simulink model "sistema_doble_pendulo"  (R2022b)
settings: Solver=VariableStepAuto  StartTime=0.0  StopTime=10  MaxStep=.00001  RelTol=1e-3
undefined symbols (not defined in the file): g, l1, l2, m1, m2
settings Model: Creator=bryan  LastModifiedBy=bryan

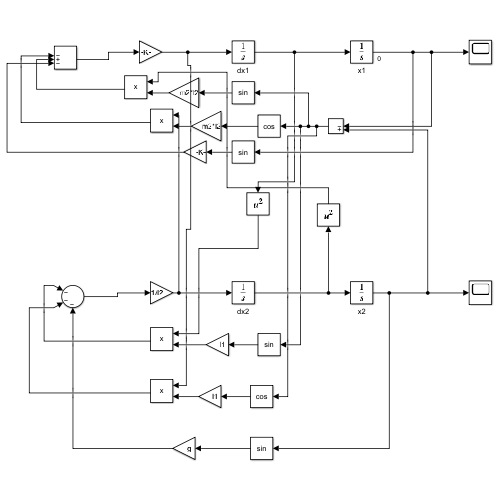
[thumbnail: Simulink's stored preview of the top-level diagram]
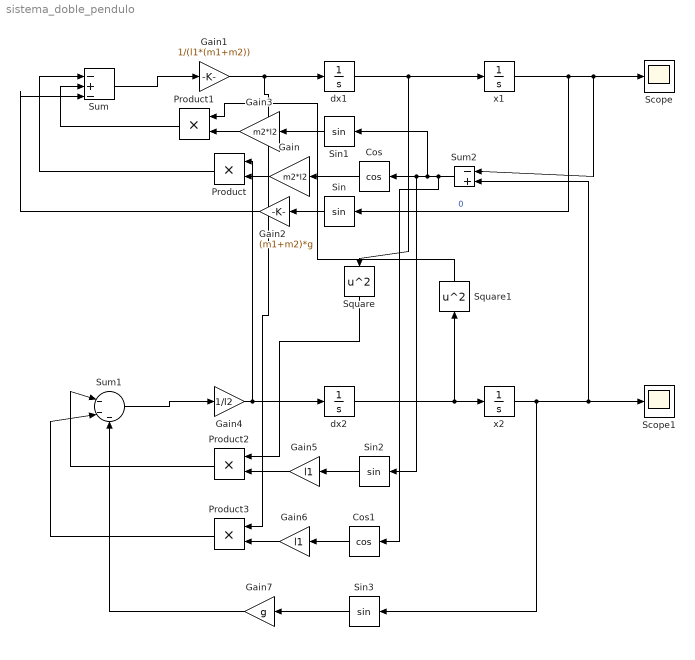
== system sistema_doble_pendulo ==
  Cos : Trigonometry  Operator=cos
  Cos1 : Trigonometry  Operator=cos
  Gain : Gain  Gain=m2*l2
  Gain1 : Gain  Gain=1/(l1*(m1+m2))
  Gain2 : Gain  Gain=(m1+m2)*g
  Gain3 : Gain  Gain=m2*l2
  Gain4 : Gain  Gain=1/l2
  Gain5 : Gain  Gain=l1
  Gain6 : Gain  Gain=l1
  Gain7 : Gain  Gain=g
  Product{,1..3} (4 alike) : Product
  Scope : Scope
  Scope1 : Scope
  Sin{,1..3} (4 alike) : Trigonometry
  Square : Math  Operator=square
  Square1 : Math  Operator=square
  Sum : Sum  Inputs=|-+-
  Sum1 : Sum  Inputs=|---
  Sum2 : Sum  Inputs=|-+
  dx1 : Integrator
  dx2 : Integrator
  x1 : Integrator
  x2 : Integrator  InitialCondition=(35*pi)/180
  wires:
  dx1/1 -> Square/1, x1/1
  Sum/1 -> Gain1/1
  Product/1 -> Sum/1
  Sin/1 -> Gain2/1
  Gain/1 -> Product/2
  Cos/1 -> Gain/1
  Gain2/1 -> Sum/3
  Sin1/1 -> Gain3/1
  Gain3/1 -> Product1/2
  Product1/1 -> Sum/2
  dx2/1 -> Square1/1, x2/1
  Gain4/1 -> dx2/1, Product/1
  Sum1/1 -> Gain4/1
  Product2/1 -> Sum1/1
  Product3/1 -> Sum1/2
  Cos1/1 -> Gain6/1
  Sin2/1 -> Gain5/1
  Gain6/1 -> Product3/2
  Gain5/1 -> Product2/2
  Sin3/1 -> Gain7/1
  Gain7/1 -> Sum1/3
  x2/1 -> Sin3/1, Sum2/2, Scope1/1
  x1/1 -> Sin/1, Sum2/1, Scope/1  "0"
  Sum2/1 -> Cos1/1, Sin1/1, Sin2/1, Cos/1
  Gain1/1 -> Product3/1, dx1/1
  Square/1 -> Product2/1
  Square1/1 -> Product1/1
